simulink model "solar_system"  (R2020a)
settings: Solver=VariableStepAuto  StartTime=0.0  StopTime=1  RelTol=1e-3
libraries: powerlib x29, powerlib_meascontrol x3, simulink x1, re_lib x1
settings Model: Creator=hp  LastModifiedBy=hp

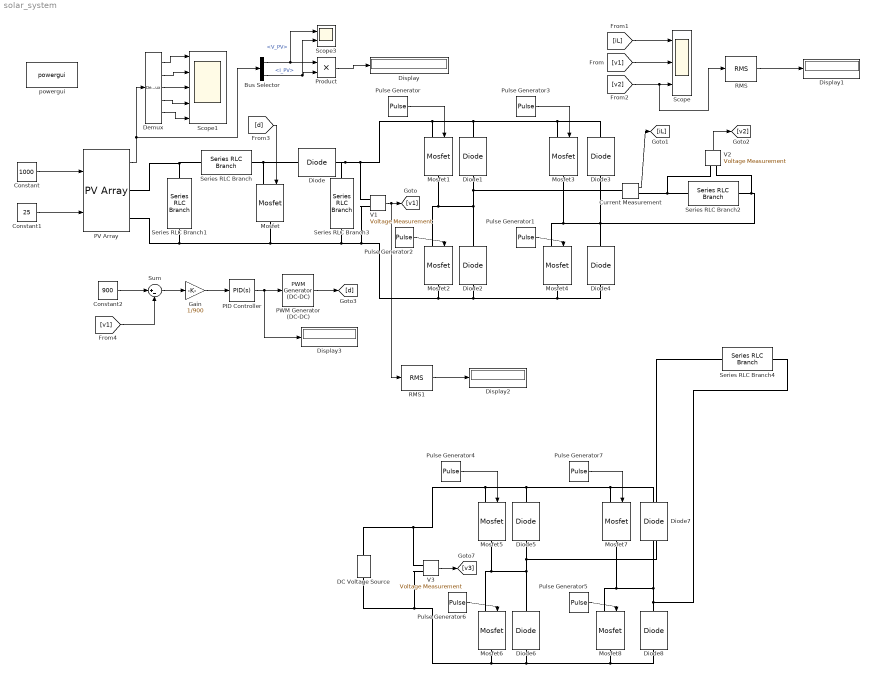
== system solar_system ==
  Bus Selector : BusSelector  OutputSignals=V_PV,I_PV
  Constant : Constant  Value=1000
  Constant1 : Constant  Value=25
  Constant2 : Constant  Value=900
  Current Measurement : powerlib/Measurements/Current Measurement  PhasorSimulation=off  OutputType=Complex  PSBequivalent=0
  DC Voltage Source : powerlib/Electrical Sources/DC Voltage Source  Amplitude=900  Measurements=None
  Demux : Demux  Outputs=5  BusSelectionMode=on
  Diode{,1..8} (9 alike) : powerlib/Power Electronics/Diode  Ron=0.001  Lon=0  Vf=0.8  IC=0  UseSnubber=0  Rs=500  Cs=250e-9  Measurements=off
  Display{,1..3} (4 alike) : Display
  Gain : Gain  Gain=1/900
  Mosfet{,1..8} (9 alike) : powerlib/Power Electronics/Mosfet  Ron=0.1  Lon=0  Rd=0.01  Vfd=0  IC=0  Rs=1e5  Cs=inf  Measurements=off
  PID Controller : simulink/Continuous/PID Controller  Controller=PID  Form=Parallel  TimeDomain=Continuous-time  UseExternalTs=off  SampleTime=-1  IntegratorMethod=Forward Euler  FilterMethod=Forward Euler  ControllerParametersSource=internal  P=-0.880412399838242  I=-108.206059793297  D=-0.00173373100099186  UseFilter=on  N=24367.8211191939  TunerSelectOption=Transfer Function Based (PID Tuner App)  InitialConditionSource=internal  InitialConditionForIntegrator=0  InitialConditionForFilter=0  DifferentiatorICPrevScaledInput=0  ExternalReset=none  TrackingMode=off  Kt=1  LimitOutput=on  UpperSaturationLimit=0.8429  LowerSaturationLimit=0.3675  LinearizeAsGain=on  AntiWindupMode=none  Kb=1  POutMin=[]  POutMax=[]  IOutMin=[]  IOutMax=[]  DOutMin=[]  DOutMax=[]  NOutMin=[]  NOutMax=[]  SumOutMin=[]  SumOutMax=[]  SaturationOutMin=[]  SaturationOutMax=[]  PParamMin=[]  PParamMax=[]  IParamMin=[]  IParamMax=[]  DParamMin=[]  DParamMax=[]  NParamMin=[]  NParamMax=[]  KbParamMin=[]  KbParamMax=[]  KtParamMin=[]  KtParamMax=[]  KbOutMin=[]  KbOutMax=[]  KtOutMin=[]  KtOutMax=[]  IntegratorOutMin=[]  IntegratorOutMax=[]  FilterOutMin=[]  FilterOutMax=[]  SumI1OutMin=[]  SumI1OutMax=[]  SumI2OutMin=[]  SumI2OutMax=[]  SumI3OutMin=[]  SumI3OutMax=[]  SumI4OutMin=[]  SumI4OutMax=[]  SumDOutMin=[]  SumDOutMax=[]  DifferentiatorOutMin=[]  DifferentiatorOutMax=[]  FilterDiffOutCoefMin=[]  FilterDiffOutCoefMax=[]  ReciprocalOutMin=[]  ReciprocalOutMax=[]  SumDenOutMin=[]  SumDenOutMax=[]  SumNumOutMin=[]  SumNumOutMax=[]  DivideOutMin=[]  DivideOutMax=[]  UdiffTsProdOutMin=[]  UdiffTsProdOutMax=[]  NTsProdOutMin=[]  NTsProdOutMax=[]  UintegralTsProdOutMin=[]  UintegralTsProdOutMax=[]  UngainTsProdOutMin=[]  UngainTsProdOutMax=[]  IntegratorContinuousStateAttributes=''  IntegratorStateMustResolveToSignalObject=off  IntegratorRTWStateStorageClass=Auto  FilterContinuousStateAttributes=''  FilterStateMustResolveToSignalObject=off  FilterRTWStateStorageClass=Auto  ParallelPVariant=InternalParameters  IdealPVariant=Disabled  IVariant=InternalParameters  DVariant=InternalParameters  IntegratorVariant=Continuous  SatVariant=Enabled  AWVariant=Passthrough  PCopyVariant=Disabled  TRVariant=Disabled  FdbkBlocksVariant=Forward  IdealPFdbkVariant=Disabled  SatFdbkVariant=Disabled  DerivativeFilterVariant=ContFilter  NVariant=InternalParameters  NCopyVariant=Disabled  FilterICVariant=InternalICsFilter  IntegratorICVariant=InternalICs  ExternalResetVariant=Disabled  TRSumVariant=Passthrough  SumFdbkVariant=Disabled  SumVariant=Sum_PID  TsampFilterVariant=InternalTs  TsampNgainVariant=Passthrough  TsampIntegralVariant=Passthrough
  PV Array : re_lib/Solar/PV Array  Npar=4  Nser=4  PlotType=array @ 1000 W/m2 & specified temperatures  S_vec="[ 1000  500  100 ]"  Temp_C_vec="[ 45 25  ]"  ModuleName=Centrosolar America BP7-315BW  PlotWhenSelected=off  Pm=315.0042  Ncell=72  Voc=45.45  Isc=8.97  Vm=37.59  Im=8.38  beta_Voc_pc=-0.349  alpha_Isc_pc=0.037001  beta_Voc=-0.15862  alpha_Isc=0.003319  IL=8.9803  I0=1.9823e-10  nI=1.0022  Rsh=237.0635  Rs=0.27147  RobustModel=off  RobustCellTemperature=25  BAL=on  Tc=1e-6  Tfilter=5e-5
  PWM Generator (DC-DC) : powerlib_meascontrol/Pulse & Signal Generators/PWM Generator (DC-DC)  Fsw=50e3  Ts=0
  Product : Product
  Pulse Generator{,1,4..5} (4 alike) : DiscretePulseGenerator  PulseType=Time based  Period=1/(50)  PulseWidth=50  PhaseDelay=0/(360*50)
  Pulse Generator{2..3,6..7} (4 alike) : DiscretePulseGenerator  PulseType=Time based  Period=1/(50)  PulseWidth=50  PhaseDelay=180/(360*50)
  RMS : powerlib_meascontrol/Measurements/RMS  TrueRMS=on  Freq=60  RMSInit=120  Ts=0
  RMS1 : powerlib_meascontrol/Measurements/RMS  TrueRMS=on  Freq=60  RMSInit=120  Ts=0
  Scope : Scope  NumInputPorts=3
  Scope1 : Scope  NumInputPorts=5
  Scope3 : Scope  NumInputPorts=2
  Series RLC Branch : powerlib/Elements/Series RLC Branch  LConnTagsString=__new0  RConnTagsString=__new0  BranchType=L  Resistance=1  Inductance=0.0021  SetiL0=off  InitialCurrent=0  Capacitance=1e-6  Setx0=off  InitialVoltage=0  Measurements=None
  Series RLC Branch1 : powerlib/Elements/Series RLC Branch  LConnTagsString=__new0  RConnTagsString=__new0  BranchType=C  Resistance=1  Inductance=1e-3  SetiL0=off  InitialCurrent=0  Capacitance=1e-6  Setx0=off  InitialVoltage=0  Measurements=None
  Series RLC Branch2 : powerlib/Elements/Series RLC Branch  LConnTagsString=__new0  RConnTagsString=__new0  BranchType=R  Resistance=181.6700  Inductance=1e-3  SetiL0=off  InitialCurrent=0  Capacitance=1e-6  Setx0=off  InitialVoltage=0  Measurements=None
  Series RLC Branch3 : powerlib/Elements/Series RLC Branch  LConnTagsString=__new0  RConnTagsString=__new0  BranchType=C  Resistance=1  Inductance=1e-3  SetiL0=off  InitialCurrent=0  Capacitance=64e-6  Setx0=off  InitialVoltage=0  Measurements=None
  Series RLC Branch4 : powerlib/Elements/Series RLC Branch  LConnTagsString=__new0  RConnTagsString=__new0  BranchType=R  Resistance=181.6700  Inductance=1e-3  SetiL0=off  InitialCurrent=0  Capacitance=1e-6  Setx0=off  InitialVoltage=0  Measurements=None
  Sum : Sum  Inputs=|+-
  V1 : powerlib/Measurements/Voltage Measurement  PhasorSimulation=off  OutputType=Complex  PSBequivalent=0
  V2 : powerlib/Measurements/Voltage Measurement  PhasorSimulation=off  OutputType=Complex  PSBequivalent=0
  V3 : powerlib/Measurements/Voltage Measurement  PhasorSimulation=off  OutputType=Complex  PSBequivalent=0
  powergui : powerlib/powergui  Priority=1  SimulationMode=Discrete  SampleTime=50e-8  frequency=60  Iterations=50  frequencyindice=0  Pbase=100e6  ErrMax=1e-4  UnitsV=kV  UnitsW=MW  buscounter=0  FunctionMessages=off  echomessages=off  EnableUseOfTLC=off  CurrentSourceSwitches=off  DisableSnubberDevices=off  DisableRonSwitches=off  DisableVfSwitches=off  DisplayEquations=off  AutomaticDiscreteSolvers=off  SolverType=Tustin/Backward Euler (TBE)  Interpol=off  ExternalGateDelay=off  methode=off  Ts=100  x0status=blocks  SPID=on  SwTol=0  HookPort=off  NonlinearTolerance=1e-4  nMaxIteration=100  ContinueOnMaxIteration=off  RestoreLinks=warning  ResistiveCurrentMeasurement=off  Frange=[0:2:500]  Ylog=off  Xlog=on  ShowGrid=off  save=off  variable=ZData  structure=0  ZoomFFT=off  StartTime=0.0  cycles=1  DisplayStyle=1  fundamental=60  FreqAxis=off  MaxFrequency=1000  frequencyindicesteady=1  RmsSteady=1  display=off
  wires:
  Constant/1 -> PV Array/1
  Constant1/1 -> PV Array/2
  PV Array/1 -> Demux/1, Bus Selector/1
  Demux/1 -> Scope1/1
  Demux/2 -> Scope1/2
  Demux/3 -> Scope1/3
  Demux/4 -> Scope1/4
  [v1] -> Scope/2
  V1/1 -> RMS1/1, [v1]
  Current Measurement/1 -> [iL]
  V2/1 -> [v2]
  [iL] -> Scope/1
  [v2] -> RMS/1, Scope/3
  [d] -> Mosfet/1
  PID Controller/1 -> Display3/1, PWM Generator (DC-DC)/1
  Gain/1 -> PID Controller/1
  Constant2/1 -> Sum/1
  Sum/1 -> Gain/1
  Demux/5 -> Scope1/5
  Pulse Generator/1 -> Mosfet1/1
  Pulse Generator1/1 -> Mosfet4/1
  Pulse Generator2/1 -> Mosfet2/1
  Pulse Generator3/1 -> Mosfet3/1
  Product/1 -> Display/1
  Bus Selector/1 -> Scope3/1, Product/1  "<V_PV>"
  Bus Selector/2 -> Scope3/2, Product/2  "<I_PV>"
  [v1] -> Sum/2
  PWM Generator (DC-DC)/1 -> [d]
  Pulse Generator5/1 -> Mosfet8/1
  V3/1 -> [v3]
  Pulse Generator6/1 -> Mosfet6/1
  Pulse Generator7/1 -> Mosfet7/1
  Pulse Generator4/1 -> Mosfet5/1
  RMS/1 -> Display1/1
  RMS1/1 -> Display2/1
  connections:
  PV Array/RConn1 -- Series RLC Branch1/LConn1 -- Series RLC Branch/LConn1
  Series RLC Branch1/RConn1 -- PV Array/RConn2 -- Diode2/LConn1 -- Diode4/LConn1 -- Mosfet4/RConn1 -- Mosfet2/RConn1 -- V1/LConn2 -- Series RLC Branch3/RConn1 -- Mosfet/RConn1
  Mosfet/LConn1 -- Diode/LConn1 -- Series RLC Branch/RConn1
  Diode/RConn1 -- V1/LConn1 -- Diode1/RConn1 -- Diode3/RConn1 -- Mosfet3/LConn1 -- Mosfet1/LConn1 -- Series RLC Branch3/LConn1
  Mosfet2/LConn1 -- Mosfet1/RConn1 -- Current Measurement/LConn1 -- Diode1/LConn1 -- Diode2/RConn1
  Diode8/RConn1 -- Series RLC Branch4/RConn1 -- Diode7/LConn1 -- Mosfet8/LConn1 -- Mosfet7/RConn1
  Diode6/RConn1 -- Mosfet5/RConn1 -- Mosfet6/LConn1 -- Series RLC Branch4/LConn1 -- Diode5/LConn1
  Mosfet8/RConn1 -- Diode8/LConn1 -- Diode6/LConn1 -- V3/LConn2 -- DC Voltage Source/LConn1 -- Mosfet6/RConn1
  Mosfet5/LConn1 -- Diode5/RConn1 -- Diode7/RConn1 -- Mosfet7/LConn1 -- DC Voltage Source/RConn1 -- V3/LConn1
  Current Measurement/RConn1 -- V2/LConn1 -- Series RLC Branch2/LConn1
  Series RLC Branch2/RConn1 -- Mosfet3/RConn1 -- Mosfet4/LConn1 -- Diode4/RConn1 -- Diode3/LConn1 -- V2/LConn2
